simulink model "EPS_Dynamic_Model"  (R2022b)
settings: Solver=VariableStepAuto  StartTime=0.0  StopTime=8  MaxStep=0.001  RelTol=1e-3
undefined symbols (not defined in the file): Br, Bs, Js, kr, ks, m, rp, sigbuilder_block
settings Model: Creator=dangm  LastModifiedBy=ASUS
settings SolverCC: AlgebraicLoopSolver=TrustRegion
settings DebuggingCC: UnconnectedInputMsg=warning  UnconnectedOutputMsg=warning  UnconnectedLineMsg=warning  SFMachineParentedDataDiag=warning
settings ModelReferenceCC: EnableRefExpFcnMdlSchedulingChecks=on

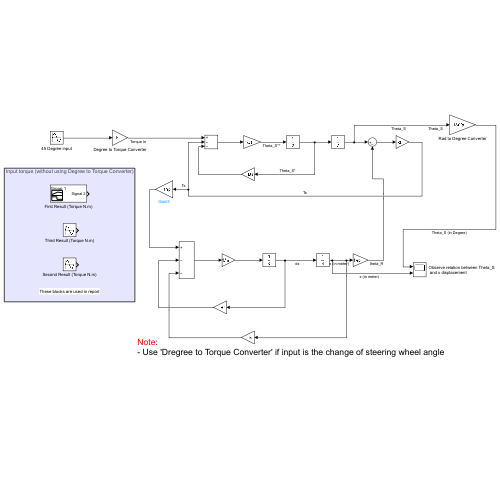
[thumbnail: Simulink's stored preview of the top-level diagram]
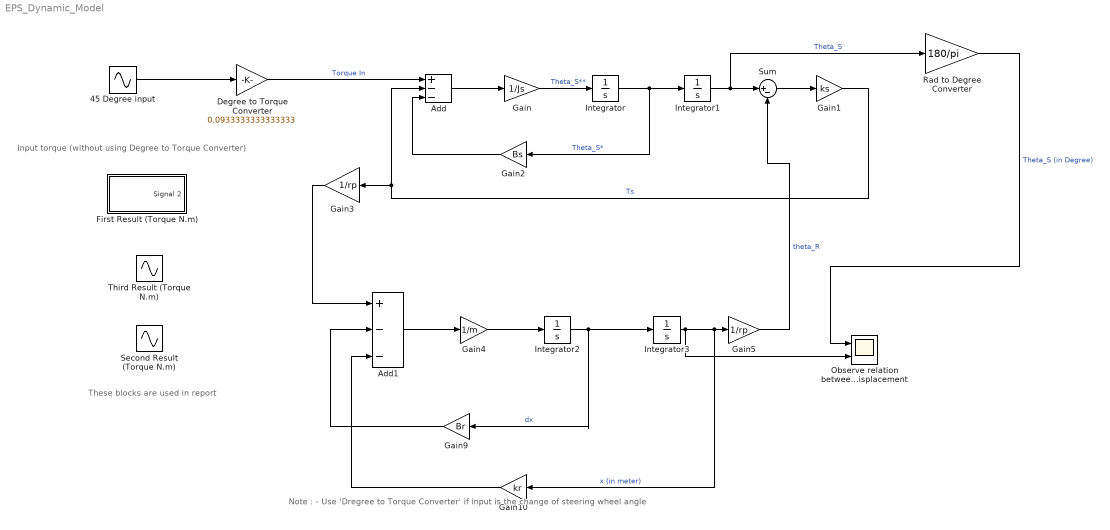
== system EPS_Dynamic_Model ==
  note: These blocks are used in report
  note: Input torque (without using Degree to Torque Converter)
  note: Note :
      | - Use 'Dregree to Torque Converter' if input is the change of steering wheel angle
  45 Degree input : Sin  Amplitude=45  SampleTime=0
  Add : Sum  Inputs=+--
  Add1 : Sum  Inputs=+--
  Degree to Torque Converter : Gain  Gain=0.0933333333333333
  First Result (Torque N.m) : Subsystem  Tag=STV Subsys  LoadFcn=sigbuilder_block('load');  StartFcn=sigbuilder_block('start');  StopFcn=sigbuilder_block('stop');  ClipboardFcn=sigbuilder_block('clipboard');  mask(Sigbuilder block){tuvar=[0:10]}
      mask help: Simulink:masks:SigbuilderBlock_MD
      mask init:
      | if ~strcmp(get_param(bdroot(gcbh),'SimulationStatus'),'stopped') tuvar = sigbuilder_block('maskInit'); end
      settings: CopyFcn=sigbuilder_block('copy');  DeleteFcn=sigbuilder_block('delete');  ModelCloseFcn=sigbuilder_block('modelClose');  PreSaveFcn=sigbuilder_block('preSave');  PauseFcn=sigbuilder_block('pause');  ContinueFcn=sigbuilder_block('continue');  NameChangeFcn=sigbuilder_block('namechange');  OpenFcn=sigbuilder_block('open',[404 117.5 550.5 362.5 ]);  CloseFcn=sigbuilder_block('close');
      mask Display: plot(0, 0, 100, 100,[2, 2, 32, 32, 2], [68, 8, 8, 68, 68],[32, 2], [38, 38], [32, 19, 2],[53, 60, 44], [32, 17, 17, 2],[16, 16, 31, 31]);txt = getActiveGroup(gcbh);text(2, 100, txt,'verticalAlignment', 'top');
  Gain : Gain  Gain=1/Js
  Gain1 : Gain  Gain=ks
  Gain10 : Gain  Gain=kr
  Gain2 : Gain  Gain=Bs
  Gain3 : Gain  Gain=1/rp
  Gain4 : Gain  Gain=1/m
  Gain5 : Gain  Gain=1/rp
  Gain9 : Gain  Gain=Br
  Integrator{,1..3} (4 alike) : Integrator
  Observe relation between Theta_S and x displacement : Scope  NumInputPorts=2
  Rad to Degree Converter : Gain  Gain=180/pi
  Second Result (Torque N.m) : Sin  Amplitude=28  SampleTime=0
  Sum : Sum  Inputs=|+-
  Third Result (Torque N.m) : Sin  Amplitude=28  Frequency=2  SampleTime=0
  wires:
  Add/1 -> Gain/1
  Gain/1 -> Integrator/1  "Theta_S**"
  Integrator/1 -> Gain2/1, Integrator1/1  "Theta_S*"
  Integrator1/1 -> Rad to Degree Converter/1, Sum/1  "Theta_S"
  Sum/1 -> Gain1/1
  Gain2/1 -> Add/3
  Gain1/1 -> Add/2, Gain3/1  "Ts"
  Gain3/1 -> Add1/1
  Add1/1 -> Gain4/1
  Gain4/1 -> Integrator2/1
  Integrator2/1 -> Gain9/1, Integrator3/1  "dx"
  Integrator3/1 -> Observe relation between Theta_S and x displacement/2, Gain10/1, Gain5/1  "x (in meter)"
  Gain5/1 -> Sum/2  "theta_R"
  Gain9/1 -> Add1/2
  Gain10/1 -> Add1/3
  Rad to Degree Converter/1 -> Observe relation between Theta_S and x displacement/1  "Theta_S (in Degree)"
  45 Degree input/1 -> Degree to Torque Converter/1
  Degree to Torque Converter/1 -> Add/1  "Torque In"

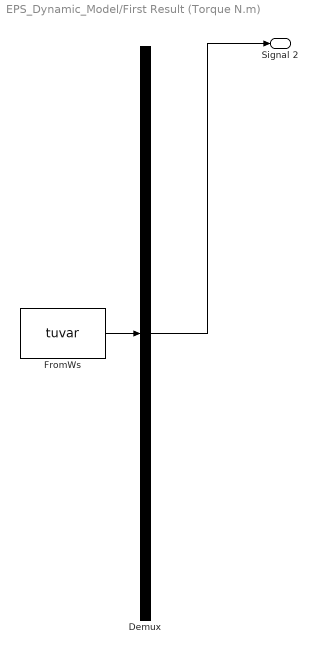
== system EPS_Dynamic_Model/First Result (Torque N.m) ==
  Demux : Demux  Tag=STV Demux  Outputs=1
      settings: DisplayOption=none
  FromWs : FromWorkspace  Tag=STV FromWs  VariableName=tuvar
      SigBuilderData=|
      | common.afterFinalStr = 'Extrapolate'
      | common.sampleTime = 0
      | dataSet.timeRange = [0 10]
      | dataSet.name = 'Group 1'
      | sbobj.Groups.Name = 'Group 1'
      | sbobj.Groups.Signals.Name = 'Signal 2'
      | sbobj.Groups.Signals.XData = [0 3 3 10]
      | sbobj.Groups.Signals.YData = [0 0 5 5]
  Signal 2 : Outport  Tag=STV Outport
  wires:
  FromWs/1 -> Demux/1
  Demux/1 -> Signal 2/1
